simulink model "Term_Simulink_wCAN"  (R2020b)
settings: Solver=ode3  StartTime=0.0  StopTime=30  FixedStep=0.002  MaxStep=1  RelTol=100e-3  EnableMultiTasking=on
model workspace (MAT data in the model file):
  der = -0.0409742647059
  integ = 3.47058823529
  prop = 3.48235294118
libraries: arduinolib x9, pid_lib x2
settings Model: SimulationMode=external  SILPILModeSetting=veronly  ExtModeTrigDuration=2  OrderedModelArguments=off  Creator=PoisonGryphon  LastModifiedBy=PoisonGryphon
settings SolverCC: InitialStep=0.2  PositivePriorityOrder=on  InsertRTBMode=Always
settings OptimizationCC: EnhancedBackFolding=on  PassReuseOutputArgsAs=Individual arguments  ZeroExternalMemoryAtStartup=off  ZeroInternalMemoryAtStartup=off  MaxStackSize=64  OptimizeBlockOrder=speed  DifferentSizesBufferReuse=on  EfficientTunableParamExpr=on
settings DebuggingCC: ParameterTunabilityLossMsg=error
settings HardwareCC: ProdBitPerInt=16  ProdBitPerPointer=16  ProdBitPerSizeT=16  ProdBitPerPtrDiffT=16  ProdLargestAtomicFloat=None  ProdWordSize=8  ProdHWDeviceType=Atmel->AVR  UseEmbeddedCoderFeatures=off  UseSimulinkCoderFeatures=off
settings SFSimCC: MATLABDynamicMemAlloc=off
settings RTWCC: Description=Embedded Coder  SystemTargetFile=ert.tlc  HardwareBoard=Arduino Mega 2560  TemplateMakefile=ert_default_tmf  RTWVerbose=off  Toolchain=Arduino AVR  BuildConfiguration=Faster Runs
settings CodeAppCC: ForceParamTrailComments=on  IgnoreCustomStorageClasses=off  MaxIdLength=95  OperatorAnnotations=on  SimulinkDataObjDesc=on  SFDataObjDesc=on  MangleLength=10  InsertBlockDesc=on
settings ERTTargetCC: SupportContinuousTime=on  SupportNonInlinedSFcns=on  SupportVariableSizeSignals=on  ExtModeStaticAllocSize=2048

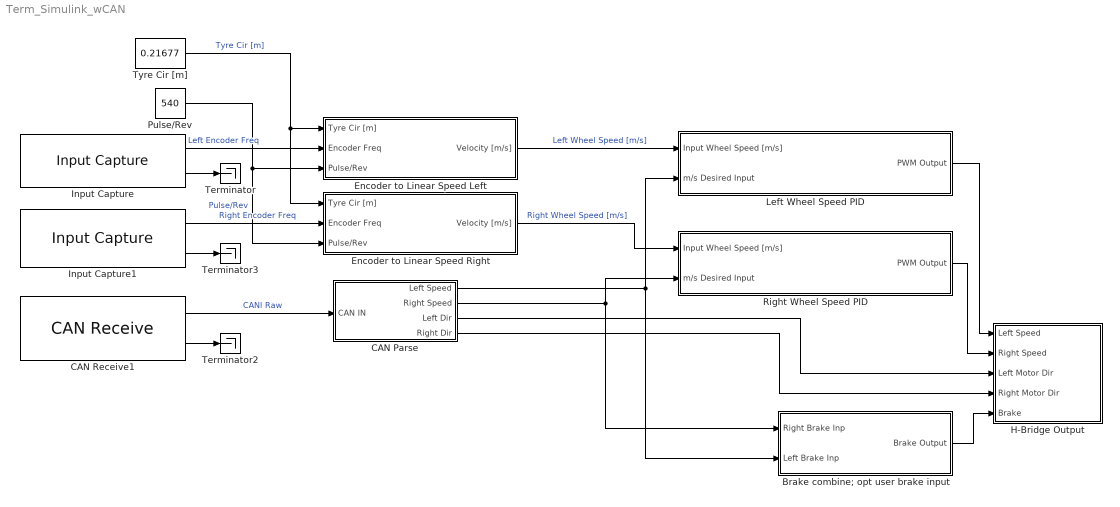
== system Term_Simulink_wCAN ==
  Brake combine; opt user brake input : Subsystem
  CAN Parse : Subsystem
  CAN Receive1 : arduinolib/CAN Receive  outputDataType=Raw data  identifierType=Standard (11-bit identifier)  messageId=hex2dec('100')  msgLength=8  SampleTime=0.1  outputError=off  outputRemote=off
      settings: SourceProductBaseCode=ARDUINO
  Encoder to Linear Speed Left : Subsystem
  Encoder to Linear Speed Right : Subsystem
  H-Bridge Output : Subsystem
  Input Capture : arduinolib/Input Capture  InputCapturePinNumber=48  SampleTime=0.002
      settings: SourceProductBaseCode=ARDUINO
  Input Capture1 : arduinolib/Input Capture  InputCapturePinNumber=49  SampleTime=0.002
      settings: SourceProductBaseCode=ARDUINO
  Left Wheel Speed PID : Subsystem
  Pulse/Rev : Constant  Value=540
  Right Wheel Speed PID : Subsystem
  Terminator : Terminator
  Terminator2 : Terminator
  Terminator3 : Terminator
  Tyre Cir [m] : Constant  Value=0.21677  OutDataTypeStr=Inherit: Inherit via back propagation
  wires:
  Input Capture/2 -> Terminator/1
  Tyre Cir [m]/1 -> Encoder to Linear Speed Right/1(Tyre Cir [m]), Encoder to Linear Speed Left/1(Tyre Cir [m])  "Tyre Cir [m]"
  Pulse/Rev/1 -> Encoder to Linear Speed Right/3(Pulse/Rev), Encoder to Linear Speed Left/3(Pulse/Rev)  "Pulse/Rev"
  Encoder to Linear Speed Left/1(Velocity [m/s]) -> Left Wheel Speed PID/1(Input Wheel Speed [m/s])  "Left Wheel Speed [m/s]"
  Left Wheel Speed PID/1(PWM Output) -> H-Bridge Output/1(Left Speed)
  Right Wheel Speed PID/1(PWM Output) -> H-Bridge Output/2(Right Speed)
  Input Capture/1 -> Encoder to Linear Speed Left/2(Encoder Freq)  "Left Encoder Freq"
  Brake combine; opt user brake input/1(Brake Output) -> H-Bridge Output/5(Brake)
  CAN Receive1/2 -> Terminator2/1
  CAN Receive1/1 -> CAN Parse/1(CAN IN)  "CANl Raw"
  Input Capture1/1 -> Encoder to Linear Speed Right/2(Encoder Freq)  "Right Encoder Freq"
  Encoder to Linear Speed Right/1(Velocity [m/s]) -> Right Wheel Speed PID/1(Input Wheel Speed [m/s])  "Right Wheel Speed [m/s]"
  Input Capture1/2 -> Terminator3/1
  CAN Parse/1(Left Speed) -> Left Wheel Speed PID/2(m/s Desired Input), Brake combine; opt user brake input/2(Left Brake Inp)
  CAN Parse/2(Right Speed) -> Brake combine; opt user brake input/1(Right Brake Inp), Right Wheel Speed PID/2(m/s Desired Input)
  CAN Parse/3(Left Dir) -> H-Bridge Output/3(Left Motor Dir)
  CAN Parse/4(Right Dir) -> H-Bridge Output/4(Right Motor Dir)

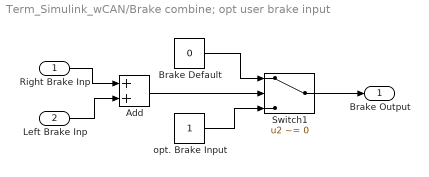
== system Term_Simulink_wCAN/Brake combine; opt user brake input ==
  Right Brake Inp : Inport
  Left Brake Inp : Inport  Port=2
  Add : Sum
  Brake Default : Constant  Value=0
  Switch1 : Switch  Criteria=u2 ~= 0
  opt. Brake Input : Constant
  Brake Output : Outport
  wires:
  Brake Default/1 -> Switch1/1
  opt. Brake Input/1 -> Switch1/3
  Right Brake Inp/1 -> Add/1
  Add/1 -> Switch1/2
  Switch1/1 -> Brake Output/1
  Left Brake Inp/1 -> Add/2

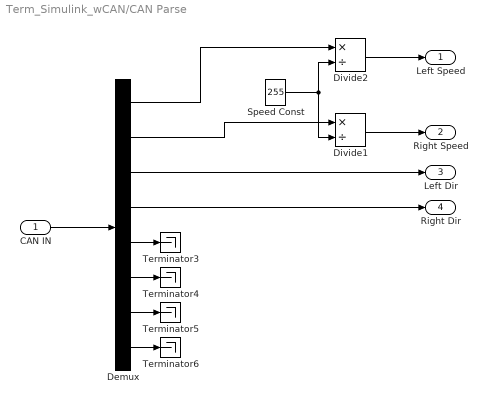
== system Term_Simulink_wCAN/CAN Parse ==
  CAN IN : Inport
  Demux : Demux  Outputs=8
  Divide1 : Product  Inputs=*/  RndMeth=Zero  SaturateOnIntegerOverflow=on
  Divide2 : Product  Inputs=*/  RndMeth=Zero  SaturateOnIntegerOverflow=on
  Speed Const : Constant  Value=255
  Terminator{3..6} (4 alike) : Terminator
  Left Speed : Outport  VectorParamsAs1DForOutWhenUnconnected=off
  Right Speed : Outport  Port=2  VectorParamsAs1DForOutWhenUnconnected=off
  Left Dir : Outport  Port=3  VectorParamsAs1DForOutWhenUnconnected=off
  Right Dir : Outport  Port=4  VectorParamsAs1DForOutWhenUnconnected=off
  wires:
  CAN IN/1 -> Demux/1
  Speed Const/1 -> Divide2/2, Divide1/2
  Demux/1 -> Divide2/1
  Demux/2 -> Divide1/1
  Demux/3 -> Left Dir/1
  Demux/4 -> Right Dir/1
  Demux/5 -> Terminator3/1
  Demux/6 -> Terminator4/1
  Demux/7 -> Terminator5/1
  Demux/8 -> Terminator6/1
  Divide2/1 -> Left Speed/1
  Divide1/1 -> Right Speed/1

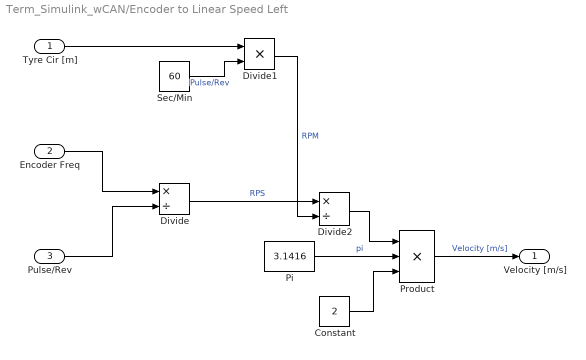
== system Term_Simulink_wCAN/Encoder to Linear Speed Left ==
  Tyre Cir [m] : Inport
  Encoder Freq : Inport  Port=2
  Pulse/Rev : Inport  Port=3
  Constant : Constant  Value=2
  Divide : Product  Inputs=*/
  Divide1 : Product  Inputs=**
  Divide2 : Product  Inputs=*/  RndMeth=Zero  SaturateOnIntegerOverflow=on
  Pi : Constant  Value=3.1416  OutDataTypeStr=Inherit: Inherit via back propagation
  Product : Product  Inputs=3
  Sec/Min : Constant  Value=60
  Velocity [m/s] : Outport
  wires:
  Constant/1 -> Product/3
  Encoder Freq/1 -> Divide/1
  Divide2/1 -> Product/1
  Pi/1 -> Product/2  "pi"
  Sec/Min/1 -> Divide1/2  "Pulse/Rev"
  Pulse/Rev/1 -> Divide/2
  Tyre Cir [m]/1 -> Divide1/1
  Product/1 -> Velocity [m/s]/1  "Velocity [m/s]"
  Divide/1 -> Divide2/1  "RPS"
  Divide1/1 -> Divide2/2  "RPM"

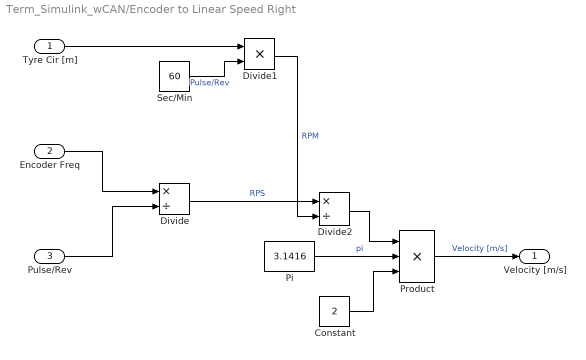
== system Term_Simulink_wCAN/Encoder to Linear Speed Right ==
  Tyre Cir [m] : Inport
  Encoder Freq : Inport  Port=2
  Pulse/Rev : Inport  Port=3
  Constant : Constant  Value=2
  Divide : Product  Inputs=*/
  Divide1 : Product  Inputs=**
  Divide2 : Product  Inputs=*/  RndMeth=Zero  SaturateOnIntegerOverflow=on
  Pi : Constant  Value=3.1416  OutDataTypeStr=Inherit: Inherit via back propagation
  Product : Product  Inputs=3
  Sec/Min : Constant  Value=60
  Velocity [m/s] : Outport
  wires:
  Constant/1 -> Product/3
  Encoder Freq/1 -> Divide/1
  Divide2/1 -> Product/1
  Pi/1 -> Product/2  "pi"
  Sec/Min/1 -> Divide1/2  "Pulse/Rev"
  Pulse/Rev/1 -> Divide/2
  Tyre Cir [m]/1 -> Divide1/1
  Product/1 -> Velocity [m/s]/1  "Velocity [m/s]"
  Divide/1 -> Divide2/1  "RPS"
  Divide1/1 -> Divide2/2  "RPM"

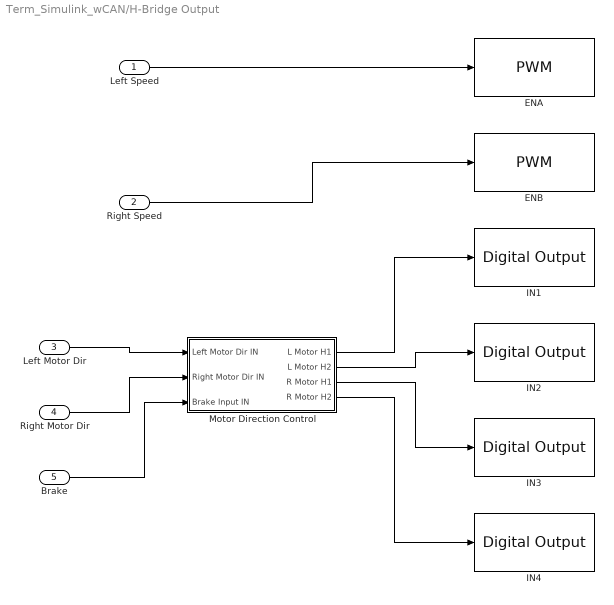
== system Term_Simulink_wCAN/H-Bridge Output ==
  Left Speed : Inport
  Right Speed : Inport  Port=2
  Left Motor Dir : Inport  Port=3
  Right Motor Dir : Inport  Port=4
  Brake : Inport  Port=5
  ENA : arduinolib/PWM  pinNumber=11  frequencyType=Default  desiredFrequency=490.2  achievableFrequency=490.2
  ENB : arduinolib/PWM  pinNumber=5  frequencyType=Default  desiredFrequency=490.2  achievableFrequency=490.2
  IN1 : arduinolib/Digital Output  pinNumber=15  Direction=output  blockPlatform=arduino
  IN2 : arduinolib/Digital Output  pinNumber=16  Direction=output  blockPlatform=arduino
  IN3 : arduinolib/Digital Output  pinNumber=17  Direction=output  blockPlatform=arduino
  IN4 : arduinolib/Digital Output  pinNumber=18  Direction=output  blockPlatform=arduino
  Motor Direction Control : Subsystem
  wires:
  Right Speed/1 -> ENB/1
  Left Motor Dir/1 -> Motor Direction Control/1(Left Motor Dir IN)
  Motor Direction Control/4(R Motor H2) -> IN4/1
  Motor Direction Control/1(L Motor H1) -> IN1/1
  Right Motor Dir/1 -> Motor Direction Control/2(Right Motor Dir IN)
  Motor Direction Control/3(R Motor H1) -> IN3/1
  Brake/1 -> Motor Direction Control/3(Brake Input IN)
  Motor Direction Control/2(L Motor H2) -> IN2/1
  Left Speed/1 -> ENA/1

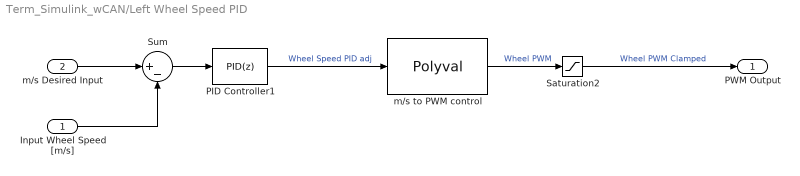
== system Term_Simulink_wCAN/Left Wheel Speed PID ==
  Input Wheel Speed [m/s] : Inport
  m/s Desired Input : Inport  Port=2
  PID Controller1 : pid_lib/PID Controller  Controller=PID  Form=Parallel  TimeDomain=Discrete-time  UseExternalTs=off  SampleTime=-1  IntegratorMethod=Forward Euler  FilterMethod=Forward Euler  ControllerParametersSource=internal  P=1.42152769348715  I=9.31457054423208  D=0.0132115900478602  UseFilter=on  N=15.4583516306973  TunerSelectOption=Transfer Function Based (PID Tuner App)  InitialConditionSource=internal  InitialConditionForIntegrator=0  InitialConditionForFilter=0  DifferentiatorICPrevScaledInput=0  ExternalReset=none  TrackingMode=off  Kt=1  LimitOutput=on  SatLimitsSource=internal  UpperSaturationLimit=5  LowerSaturationLimit=-5  LinearizeAsGain=on  AntiWindupMode=none  Kb=1  POutMin=[]  POutMax=[]  IOutMin=[]  IOutMax=[]  DOutMin=[]  DOutMax=[]  NOutMin=[]  NOutMax=[]  SumOutMin=[]  SumOutMax=[]  SaturationOutMin=[]  SaturationOutMax=[]  PParamMin=[]  PParamMax=[]  IParamMin=[]  IParamMax=[]  DParamMin=[]  DParamMax=[]  NParamMin=[]  NParamMax=[]  KbParamMin=[]  KbParamMax=[]  KtParamMin=[]  KtParamMax=[]  KbOutMin=[]  KbOutMax=[]  KtOutMin=[]  KtOutMax=[]  IntegratorOutMin=[]  IntegratorOutMax=[]  FilterOutMin=[]  FilterOutMax=[]  SumI1OutMin=[]  SumI1OutMax=[]  SumI2OutMin=[]  SumI2OutMax=[]  SumI3OutMin=[]  SumI3OutMax=[]  SumI4OutMin=[]  SumI4OutMax=[]  SumDOutMin=[]  SumDOutMax=[]  DifferentiatorOutMin=[]  DifferentiatorOutMax=[]  FilterDiffOutCoefMin=[]  FilterDiffOutCoefMax=[]  ReciprocalOutMin=[]  ReciprocalOutMax=[]  SumDenOutMin=[]  SumDenOutMax=[]  SumNumOutMin=[]  SumNumOutMax=[]  DivideOutMin=[]  DivideOutMax=[]  UdiffTsProdOutMin=[]  UdiffTsProdOutMax=[]  NTsProdOutMin=[]  NTsProdOutMax=[]  UintegralTsProdOutMin=[]  UintegralTsProdOutMax=[]  UngainTsProdOutMin=[]  UngainTsProdOutMax=[]  IntegratorContinuousStateAttributes=''  IntegratorStateMustResolveToSignalObject=off  IntegratorRTWStateStorageClass=Auto  FilterContinuousStateAttributes=''  FilterStateMustResolveToSignalObject=off  FilterRTWStateStorageClass=Auto  ParallelPVariant=InternalParameters  IdealPVariant=Disabled  IVariant=InternalParameters  DVariant=InternalParameters  IntegratorVariant=Discrete  SatVariant=Enabled  AWVariant=Passthrough  PCopyVariant=Disabled  TRVariant=Disabled  FdbkBlocksVariant=Forward  IdealPFdbkVariant=Disabled  SatFdbkVariant=Disabled  DerivativeFilterVariant=ForwardEulerFilter  NVariant=InternalParameters  NCopyVariant=Disabled  FilterICVariant=InternalICsFilter  IntegratorICVariant=InternalICs  ExternalResetVariant=Disabled  TRSumVariant=Passthrough  SumFdbkVariant=Disabled  SumVariant=Sum_PID  TsampFilterVariant=InternalTs  TsampNgainVariant=Passthrough  TsampIntegralVariant=Passthrough  ExternalSaturationOutDataTypeStr=Inherit: Same as second input
  Saturation2 : Saturate  UpperLimit=255  LowerLimit=0
  Sum : Sum  Inputs=|+-
  m/s to PWM control : Polyval  Coefs=[142.48, 104.93, 19.758]
  PWM Output : Outport
  wires:
  Input Wheel Speed [m/s]/1 -> Sum/2
  Sum/1 -> PID Controller1/1
  PID Controller1/1 -> m/s to PWM control/1  "Wheel Speed PID adj"
  m/s Desired Input/1 -> Sum/1
  m/s to PWM control/1 -> Saturation2/1  "Wheel PWM"
  Saturation2/1 -> PWM Output/1  "Wheel PWM Clamped"

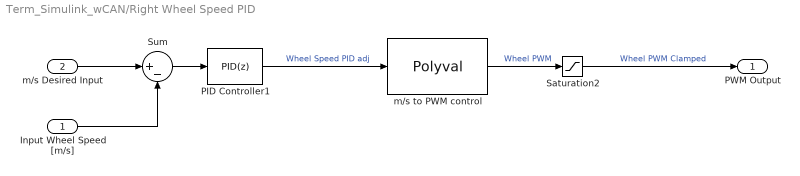
== system Term_Simulink_wCAN/Right Wheel Speed PID ==
  Input Wheel Speed [m/s] : Inport
  m/s Desired Input : Inport  Port=2
  PID Controller1 : pid_lib/PID Controller  Controller=PID  Form=Parallel  TimeDomain=Discrete-time  UseExternalTs=off  SampleTime=-1  IntegratorMethod=Forward Euler  FilterMethod=Forward Euler  ControllerParametersSource=internal  P=1.42152769348715  I=9.31457054423208  D=0.0132115900478602  UseFilter=on  N=15.4583516306973  TunerSelectOption=Transfer Function Based (PID Tuner App)  InitialConditionSource=internal  InitialConditionForIntegrator=0  InitialConditionForFilter=0  DifferentiatorICPrevScaledInput=0  ExternalReset=none  TrackingMode=off  Kt=1  LimitOutput=on  SatLimitsSource=internal  UpperSaturationLimit=5  LowerSaturationLimit=-5  LinearizeAsGain=on  AntiWindupMode=none  Kb=1  POutMin=[]  POutMax=[]  IOutMin=[]  IOutMax=[]  DOutMin=[]  DOutMax=[]  NOutMin=[]  NOutMax=[]  SumOutMin=[]  SumOutMax=[]  SaturationOutMin=[]  SaturationOutMax=[]  PParamMin=[]  PParamMax=[]  IParamMin=[]  IParamMax=[]  DParamMin=[]  DParamMax=[]  NParamMin=[]  NParamMax=[]  KbParamMin=[]  KbParamMax=[]  KtParamMin=[]  KtParamMax=[]  KbOutMin=[]  KbOutMax=[]  KtOutMin=[]  KtOutMax=[]  IntegratorOutMin=[]  IntegratorOutMax=[]  FilterOutMin=[]  FilterOutMax=[]  SumI1OutMin=[]  SumI1OutMax=[]  SumI2OutMin=[]  SumI2OutMax=[]  SumI3OutMin=[]  SumI3OutMax=[]  SumI4OutMin=[]  SumI4OutMax=[]  SumDOutMin=[]  SumDOutMax=[]  DifferentiatorOutMin=[]  DifferentiatorOutMax=[]  FilterDiffOutCoefMin=[]  FilterDiffOutCoefMax=[]  ReciprocalOutMin=[]  ReciprocalOutMax=[]  SumDenOutMin=[]  SumDenOutMax=[]  SumNumOutMin=[]  SumNumOutMax=[]  DivideOutMin=[]  DivideOutMax=[]  UdiffTsProdOutMin=[]  UdiffTsProdOutMax=[]  NTsProdOutMin=[]  NTsProdOutMax=[]  UintegralTsProdOutMin=[]  UintegralTsProdOutMax=[]  UngainTsProdOutMin=[]  UngainTsProdOutMax=[]  IntegratorContinuousStateAttributes=''  IntegratorStateMustResolveToSignalObject=off  IntegratorRTWStateStorageClass=Auto  FilterContinuousStateAttributes=''  FilterStateMustResolveToSignalObject=off  FilterRTWStateStorageClass=Auto  ParallelPVariant=InternalParameters  IdealPVariant=Disabled  IVariant=InternalParameters  DVariant=InternalParameters  IntegratorVariant=Discrete  SatVariant=Enabled  AWVariant=Passthrough  PCopyVariant=Disabled  TRVariant=Disabled  FdbkBlocksVariant=Forward  IdealPFdbkVariant=Disabled  SatFdbkVariant=Disabled  DerivativeFilterVariant=ForwardEulerFilter  NVariant=InternalParameters  NCopyVariant=Disabled  FilterICVariant=InternalICsFilter  IntegratorICVariant=InternalICs  ExternalResetVariant=Disabled  TRSumVariant=Passthrough  SumFdbkVariant=Disabled  SumVariant=Sum_PID  TsampFilterVariant=InternalTs  TsampNgainVariant=Passthrough  TsampIntegralVariant=Passthrough  ExternalSaturationOutDataTypeStr=Inherit: Same as second input
  Saturation2 : Saturate  UpperLimit=255  LowerLimit=0
  Sum : Sum  Inputs=|+-
  m/s to PWM control : Polyval  Coefs=[142.48, 104.93, 19.758]
  PWM Output : Outport
  wires:
  Input Wheel Speed [m/s]/1 -> Sum/2
  Sum/1 -> PID Controller1/1
  PID Controller1/1 -> m/s to PWM control/1  "Wheel Speed PID adj"
  m/s Desired Input/1 -> Sum/1
  m/s to PWM control/1 -> Saturation2/1  "Wheel PWM"
  Saturation2/1 -> PWM Output/1  "Wheel PWM Clamped"

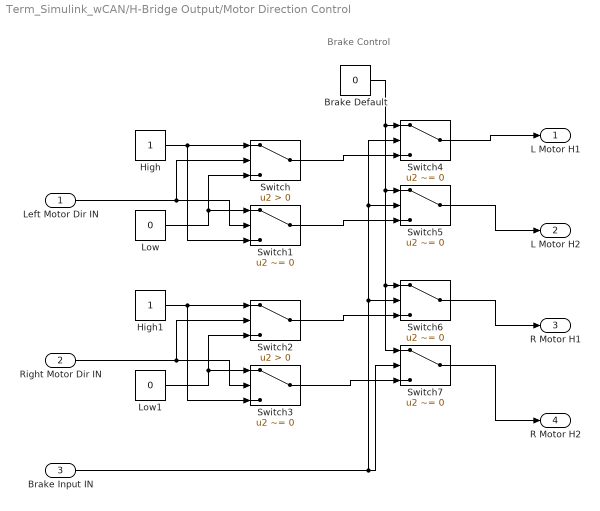
== system Term_Simulink_wCAN/H-Bridge Output/Motor Direction Control ==
  note: Brake Control
  Left Motor Dir IN : Inport
  Right Motor Dir IN : Inport  Port=2
  Brake Input IN : Inport  Port=3
  Brake Default : Constant  Value=0
  High : Constant
  High1 : Constant
  Low : Constant  Value=0
  Low1 : Constant  Value=0
  Switch : Switch  Criteria=u2 > Threshold
  Switch{1,3..7} (6 alike) : Switch  Criteria=u2 ~= 0
  Switch2 : Switch  Criteria=u2 > Threshold
  L Motor H1 : Outport
  L Motor H2 : Outport  Port=2
  R Motor H1 : Outport  Port=3
  R Motor H2 : Outport  Port=4
  wires:
  Low/1 -> Switch1/1, Switch/3
  High/1 -> Switch/1, Switch1/3
  Left Motor Dir IN/1 -> Switch1/2, Switch/2
  Right Motor Dir IN/1 -> Switch3/2, Switch2/2
  Low1/1 -> Switch3/1, Switch2/3
  High1/1 -> Switch2/1, Switch3/3
  Switch4/1 -> L Motor H1/1
  Switch5/1 -> L Motor H2/1
  Switch6/1 -> R Motor H1/1
  Switch7/1 -> R Motor H2/1
  Switch/1 -> Switch4/3
  Switch3/1 -> Switch7/3
  Brake Input IN/1 -> Switch4/2, Switch5/2, Switch6/2, Switch7/2
  Switch2/1 -> Switch6/3
  Brake Default/1 -> Switch7/1, Switch6/1, Switch5/1, Switch4/1
  Switch1/1 -> Switch5/3
